simulink model "robocar_pp"  (R2024b)
settings: Solver=FixedStepAuto  StartTime=0  StopTime=60  FixedStep=0.001  RelTol=1e-3
undefined symbols (not defined in the file or in its folder): base_wheel
libraries: robotmobilelib x1, robotalgslib x1
settings Model: Creator=saucesaft  LastModifiedBy=saucesaft
settings OptimizationCC: DefaultParameterBehavior=Inlined  UseDivisionForNetSlopeComputation=on  GainParamInheritBuiltInType=on  UseFloatMulNetSlope=on  InlineInvariantSignals=on  PassReuseOutputArgsAs=Individual arguments  ZeroExternalMemoryAtStartup=off  ZeroInternalMemoryAtStartup=off  NoFixptDivByZeroProtection=on  EfficientFloat2IntCast=on  LifeSpan=1  OptimizeBlockOrder=speed  DifferentSizesBufferReuse=on  EfficientTunableParamExpr=on
settings DebuggingCC: ParameterTunabilityLossMsg=error  SFUnexpectedBacktrackingDiag=warning  SFNoUnconditionalDefaultTransitionDiag=warning
settings HardwareCC: ProdBitPerPointer=32  ProdBitPerSizeT=32  ProdBitPerPtrDiffT=32  ProdLargestAtomicInteger=Long  ProdLargestAtomicFloat=Double  ProdWordSize=32  ProdLongLongMode=on  ProdHWDeviceType=ARM Compatible->ARM Cortex-M
settings SFSimCC: MATLABDynamicMemAlloc=off
settings RTWCC: Description=Embedded Coder  SystemTargetFile=ert.tlc  TemplateMakefile=ert_default_tmf  GenerateReport=on  BuildConfiguration=Debug  LaunchReport=on
settings CodeAppCC: ForceParamTrailComments=on  IgnoreCustomStorageClasses=off  OperatorAnnotations=on  SimulinkDataObjDesc=on  SFDataObjDesc=on  CustomSymbolStrGlobalVar=rt$N$M  CustomSymbolStrType=$N$M  CustomSymbolStrFcn=$N$M$F  CustomSymbolStrMacro=$N$M  InsertBlockDesc=on  EnableCustomComments=on
settings ERTTargetCC: TargetLangStandard=C99 (ISO)  GenerateSampleERTMain=on  IncludeMdlTerminateFcn=off  CombineSignalStateStructs=on  SupportAbsoluteTime=off  SupportComplex=off  SupportContinuousTime=on  SupportNonInlinedSFcns=on  ERTCustomFileTemplate=example_file_process.tlc  ERTFilePackagingFormat=CompactWithDataFile

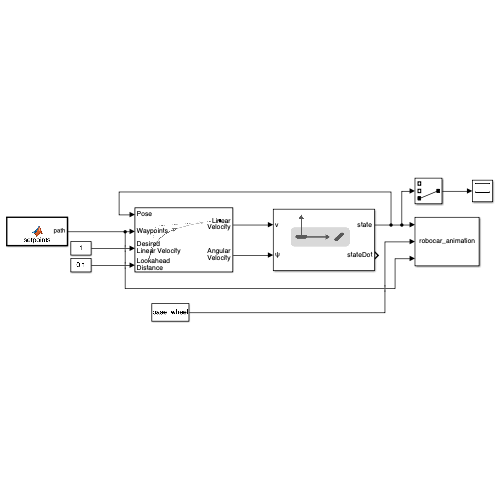
[thumbnail: Simulink's stored preview of the top-level diagram]
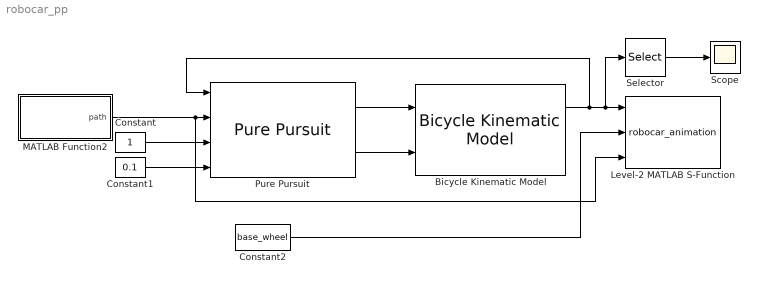
== system robocar_pp ==
  Bicycle Kinematic Model : robotmobilelib/Bicycle Kinematic Model  VehicleInputs=Vehicle Speed & Steering Angle  WheelBase=base_wheel  VehicleSpeedRange=[-inf inf]  MaxSteeringAngle=pi/4  InitialState=[0, 0, 0]  SimulateUsing=Interpreted execution
  Constant : Constant
  Constant1 : Constant  Value=0.1
  Constant2 : Constant  Value=base_wheel
  Level-2 MATLAB S-Function : M-S-Function  FunctionName=robocar_animation
  MATLAB Function2 : MATLAB Function  TreatAsAtomicUnit=on
  Pure Pursuit : robotalgslib/Pure Pursuit  DesiredLinearVelocityPort=on  DesiredLinearVelocity=0.5  MaxAngularVelocity=1.0  LookaheadDistancePort=on  LookaheadDistance=1  TargetDirPort=off  SimulateUsing=Code generation
      settings: LibrarySourceBlock=robotmobilelib/Pure Pursuit
  Scope : Scope
  Selector : Selector  InputPortWidth=3  IndexOptions=Index vector (dialog)  Indices=3  OutputSizes=1
  wires:
  MATLAB Function2/1(path) -> Level-2 MATLAB S-Function/3, Pure Pursuit/2
  Bicycle Kinematic Model/1 -> Selector/1, Level-2 MATLAB S-Function/1, Pure Pursuit/1
  Constant1/1 -> Pure Pursuit/4
  Constant/1 -> Pure Pursuit/3
  Pure Pursuit/1 -> Bicycle Kinematic Model/1
  Pure Pursuit/2 -> Bicycle Kinematic Model/2
  Constant2/1 -> Level-2 MATLAB S-Function/2
  Selector/1 -> Scope/1

== matlab function robocar_pp/MATLAB Function2 ==
  data: path output
function path  = setpoints
    x = [4  6 8  10];
    y = [5 -5 5  -5];
    path = [x; y]';
end
